simulink model "Singlephasefullwaverectifiercircuit"  (R2023a)
settings: Solver=VariableStepAuto  StartTime=0.0  StopTime=0.1  MaxStep=1e-4  RelTol=1e-3
libraries: spsThyristorLib x4, spsACVoltageSourceLib x1, spsMultimeterLib x1, spsSeriesRLCBranchLib x1, sps_lib x1
settings Model: Creator=ly frienk  LastModifiedBy=ly frienk

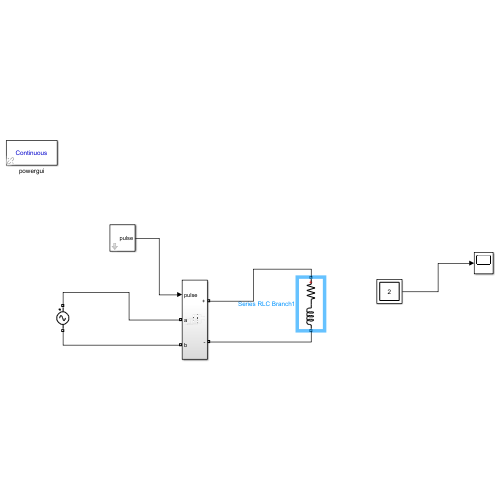
[thumbnail: Simulink's stored preview of the top-level diagram]
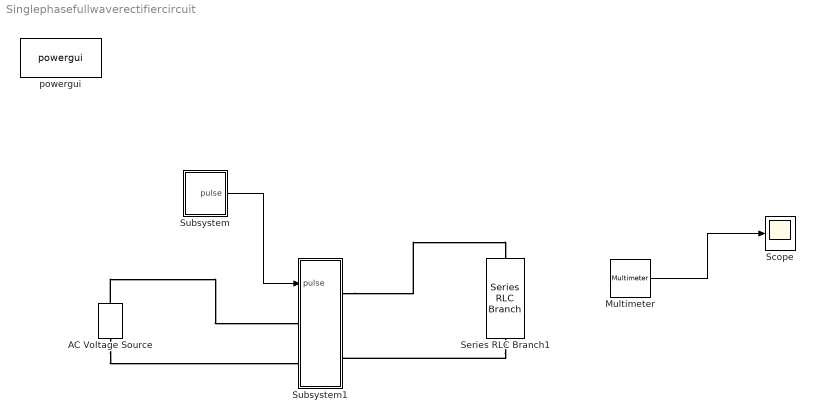
== system Singlephasefullwaverectifiercircuit ==
  AC Voltage Source : spsACVoltageSourceLib/AC Voltage Source  Amplitude=220*sqrt(2)  Phase=0  Frequency=50  SampleTime=0  Measurements=None  BusType=swing  Pref=10e3  Qref=0  Qmin=-inf  Qmax=+inf
  Multimeter : spsMultimeterLib/Multimeter  L=2  sel=[1 2]  yselected={}  Gain=[1 1]  OutputType=Complex  PlotAtSimulationStop=off  PhasorSimulation=off
  Scope : Scope
  Series RLC Branch1 : spsSeriesRLCBranchLib/Series RLC Branch  LConnTagsString=__new0  RConnTagsString=__new0  BranchType=RL  Resistance=10  Inductance=1e-3  SetiL0=off  InitialCurrent=0  Capacitance=1e-6  Setx0=off  InitialVoltage=0  Measurements=Branch voltage and current
  Subsystem : Subsystem  mask{freq=50, algha=60}
      mask prompts: freq "grid frequency"
      mask DialogControl ParameterGroupVar Prompt: 参数
  Subsystem1 : Subsystem
  powergui : sps_lib/powergui  Priority=1  SimulationMode=Continuous  SampleTime=50e-6  frequency=60  Iterations=50  frequencyindice=50  Pbase=100e6  ErrMax=1e-4  UnitsV=kV  UnitsW=MW  buscounter=0  FunctionMessages=off  echomessages=off  EnableUseOfTLC=off  CurrentSourceSwitches=off  DisableSnubberDevices=off  DisableRonSwitches=off  DisableVfSwitches=off  DisplayEquations=off  AutomaticDiscreteSolvers=off  SolverType=Tustin/Backward Euler (TBE)  Interpol=off  ExternalGateDelay=off  methode=off  Ts=100  x0status=blocks  SPID=on  SwTol=0  HookPort=off  NonlinearTolerance=1e-4  nMaxIteration=100  ContinueOnMaxIteration=off  RestoreLinks=warning  ResistiveCurrentMeasurement=off  Frange=[0:2:500]  Ylog=off  Xlog=on  ShowGrid=off  save=off  variable=ZData  structure=0  ZoomFFT=off  StartTime=0.0  cycles=1  DisplayStyle=1  fundamental=60  FreqAxis=off  MaxFrequency=1000  frequencyindicesteady=1  RmsSteady=1  display=off
  wires:
  Multimeter/1 -> Scope/1
  Subsystem/1(pulse) -> Subsystem1/1(pulse)
  connections:
  Subsystem1/RConn1 -- Series RLC Branch1/LConn1
  AC Voltage Source/RConn1 -- Subsystem1/LConn1
  AC Voltage Source/LConn1 -- Subsystem1/LConn2
  Series RLC Branch1/RConn1 -- Subsystem1/RConn2

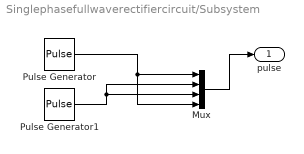
== system Singlephasefullwaverectifiercircuit/Subsystem ==
  Mux : Mux
  Pulse Generator : DiscretePulseGenerator  PulseType=Time based  Period=1/freq  PulseWidth=5  PhaseDelay=algha/360*(1/freq)
  Pulse Generator1 : DiscretePulseGenerator  PulseType=Time based  Period=1/freq  PulseWidth=5  PhaseDelay=(algha+180)/360*(1/freq)
  pulse : Outport
  wires:
  Pulse Generator/1 -> Mux/4, Mux/1
  Pulse Generator1/1 -> Mux/2, Mux/3
  Mux/1 -> pulse/1

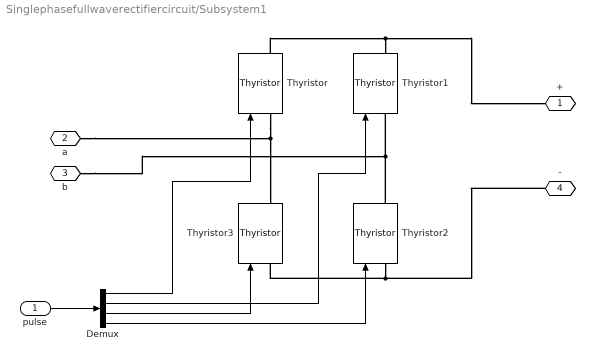
== system Singlephasefullwaverectifiercircuit/Subsystem1 ==
  pulse : Inport
  Demux : Demux
  Thyristor{,1..3} (4 alike) : spsThyristorLib/Thyristor  Ron=0.001  Lon=0  Vf=0.8  IC=0  Rs=500  Cs=250e-9  Measurements=on
  + : PMIOPort  Side=Right
  a : PMIOPort  Port=2  Side=Left
  b : PMIOPort  Port=3  Side=Left
  - : PMIOPort  Port=4  Side=Right
  wires:
  pulse/1 -> Demux/1
  Demux/1 -> Thyristor/1
  Demux/2 -> Thyristor1/1
  Demux/3 -> Thyristor3/1
  Demux/4 -> Thyristor2/1
  connections:
  Thyristor/LConn1 -- Thyristor3/RConn1 -- a/RConn1
  Thyristor/RConn1 -- Thyristor1/RConn1 -- +/RConn1
  Thyristor2/RConn1 -- b/RConn1 -- Thyristor1/LConn1
  Thyristor2/LConn1 -- -/RConn1 -- Thyristor3/LConn1
